simulink model "Backhoe_TiltCyl_Valve_Variants"  (R2020b)
settings: Solver=ode23t  StartTime=0.0  StopTime=60  MaxStep=0.01  RelTol=1e-3  EnableMultiTasking=on
PreLoadFcn:
  | Abstract=Simulink.Variant('ValveType4way==1');
  | Spool=Simulink.Variant('ValveType4way==2');
  | Nozzle_Center=Simulink.Variant('ValveType4way==3');
  | Nozzle_Feedback=Simulink.Variant('ValveType4way==4');
  | ValveType4way = 1;
  | 
  | warning('off','Simulink:Commands:LoadMdlParameterizedLink');
PostLoadFcn:
  | warning off Simulink:Engine:UsingDefaultMaxStepSize
  | warning off Simulink:blocks:MatchingFromNotFound
  | warning off Simulink:Engine:SaveWithParameterizedLinks_Warning
  | warning off Simulink:Engine:SolverMinStepNonlinearIterWarnForDAE
  | warning off Simulink:Commands:SetParamLinkChangeWarn
model workspace (MAT data in the model file):
  cylinderGray = [0.6 0.6 0.6]
  darkOrange = [0.8 0.5 0]
  glassBlue = [0.2 0.2 1]
  gray = [0.3 0.3 0.3]
  orange = [0.8 0.65 0]
  pistonGray = [0.4 0.4 0.4]
  rhoGlass = 2500
  rhoRubber = 1500
  rhoSteel = 7800
  tireBlack = [0.1 0.1 0.1]
  wheelGray = [0.6 0.6 0.6]
  yellow = [0.8 0.8 0]
undefined symbols (not defined in the file): BH_Param, sigbuilder_block, X, Y, Z
libraries: sm_lib x54, fl_lib x16, Backhoe_Lib x15, nesl_utility x8, sh_lib x6, Custom_Valve_Variants_Lib x3
(part 1 of 3)
CloseFcn:
  | try,close(h1_Backhoe_TiltCyl_Valve_Variants),end
  | clear h1_Backhoe_TiltCyl_Valve_Variants
  | try,close(h2_Backhoe_TiltCyl_Valve_Variants),end
  | clear h2_Backhoe_TiltCyl_Valve_Variants
  | try,close(h3_Backhoe_TiltCyl_Valve_Variants),end
  | clear h3_Backhoe_TiltCyl_Valve_Variants
  | try,close(h4_Backhoe_TiltCyl_Valve_Variants),end
  | clear h4_Backhoe_TiltCyl_Valve_Variants
  | 
  | clear simlog_Backhoe_TiltCyl_Valve_Variants
  | clear logsout_simlog_Backhoe_TiltCyl_Valve_Variants
Description:
  | Backhoe with Custom Valve
  | 
  | Copyright 2014-2020 The MathWorks, Inc.
settings Model: Creator=smiller  LastModifiedBy=smiller
settings DataIOCC: LimitDataPoints=on  SaveFormat=Array  ReturnWorkspaceOutputs=off
settings OptimizationCC: ExpressionDepthLimit=2147483647  LifeSpan=inf
settings DebuggingCC: UnderspecifiedInitializationDetection=Classic  MergeDetectMultiDrivingBlocksExec=none  SolverPrmCheckMsg=warning  AllowSymbolicDim=off  StateNameClashWarn=warning  PregeneratedLibrarySubsystemCodeDiagnostic=none  SFUnexpectedBacktrackingDiag=warning  SFNoUnconditionalDefaultTransitionDiag=warning  SFExecutionAtInitializationDiag=none  ArithmeticOperatorsInVariantConditions=warning
settings HardwareCC: ProdBitPerPointer=32  ProdBitPerSizeT=32  ProdBitPerPtrDiffT=32  ProdLargestAtomicFloat=None  ProdIntDivRoundTo=Undefined  ProdEndianess=Unspecified  ProdWordSize=32  ProdHWDeviceType=32-bit Generic
settings ModelReferenceCC: PropagateSignalLabelsOutOfModel=off
settings SFSimCC: SimUseLocalCustomCode=off  CustomCodeUndefinedFunction=UseInterfaceOnly
settings RTWCC: RTWUseLocalCustomCode=off
settings CodeAppCC: StateflowObjectComments=on
settings GRTTargetCC: TargetLangStandard=C89/C90 (ANSI)
settings ConfigComp: CovMetricSettings=dw  CovSaveCumulativeToWorkspaceVar=on  CovSaveSingleToWorkspaceVar=on  CovExternalEMLEnable=off  CovSFcnEnable=off
settings SimscapeCC: SimscapeNormalizeSystem=off  SimscapeLogType=all  SimscapeLogName=simlog_Backhoe_TiltCyl_Valve_Variants  SimscapeLogDataHistory=10000
settings ConfigurationSet: Description=SimMechanics 2G
settings ExplorerConfigSet: InternalSimMechanicsExplorerSettings="<ExplorerConfiguration><canonicalview>default</canonicalview><AnimationSetting><BasePlaybackSpeed>1.0</BasePlaybackSpeed><PlaybackSpeedFactor>1.0</PlaybackSpeedFactor></AnimationSetting><TilePanel><TileInfo><Tiles Columns=\"1\" Count=\"1\" Rows=\"1\"><Column Weight=\"1\"/><Row Weight=\"1\"/><Tile Height=\"1\" Width=\"1\" X=\"0\" Y=\"0\"/></Tiles></TileInfo><SceneInfo><SceneViewer><BGColor><R>1</R><G>1</G><B>1</B></BGColor><Camera><DoPerspective>off</DoPerspective><Position><X>0.528725759523142269</X><Y>-5.20390358957664034</Y><Z>-12.0546820877544469</Z></Position><Center><X>2.55521134765160207</X><Y>-1.1721933566146352</Y><Z>-0.0122773925518812436</Z></Center><Up><X>0.814497762035467865</X><Y>-0.577432689239198105</Y><Z>0.0562573109666866522</Z></Up><ViewLimDist>1</ViewLimDist><YLim>4.64006309682449647</YLim><XLim>7.37103468240321025</XLim></Camera></SceneViewer></SceneInfo></TilePanel><MechEditorPanel><Cameras/><GfxPanelCameraMap/><VideoCreator><PlaybackSpeedRatio>1.0</PlaybackSpeedRatio><FrameRate>30</FrameRate><VideoFormat>Motion JPEG AVI</VideoFormat><FrameSize>auto</FrameSize></VideoCreator></MechEditorPanel></ExplorerConfiguration>"

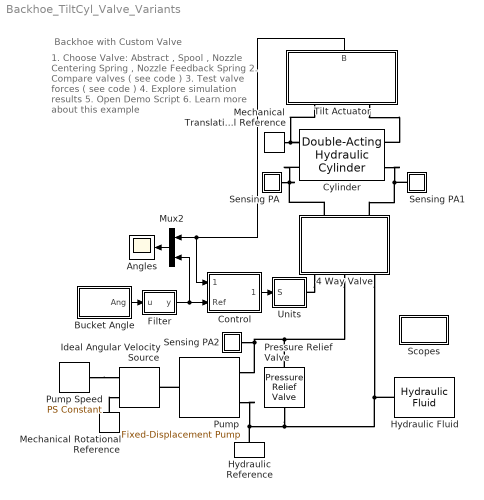
== system Backhoe_TiltCyl_Valve_Variants ==
  note: 1. Choose Valve: Abstract , Spool ,
      | Nozzle Centering Spring ,
      | Nozzle Feedback Spring
      | 2. Compare valves ( see code )
      | 3. Test valve forces ( see code )
      | 4. Explore simulation results
      | 5. Open Demo Script
      | 6. Learn more about this example
  note: Backhoe with Custom Valve
  4 Way Valve : Subsystem  InitFcn=|  BlockChoice=Servovalve_Flapper  Variant=on  mask(Four-Way Servovalve, Customizable){valvetype=Abstract, orifice_width=24.5, max_spool_travel=0.005, x0_orifice_PA=-1e-4, x0_orifice_PB=-1e-4, x0_orifice_AT=-1e-4, x0_orifice_BT=-1e-4, spool_mass=0.124, spool_damping=162, spool_rad_clear=0.05, spool_hyd_frc=Enable, x0_nozzle=0.5, max_nozzle_area=3.14, pump_spool_orifice_area=1, act_gain=250*10, act_timeconstant=1e-2, act_saturation=0.3}
      | %temp_maskObj = Simulink.Mask.get(gcb);
      | %temp_vt_h = temp_maskObj.getParameter('valvetype');
      | %set_param(gcb,'valvetype',temp_vt_h.TypeOptions{ValveType4way});
      mask prompts: valvetype "Valve Type"; orifice_width "Orifice Width (mm):"; max_spool_travel "Max Orifice Length (m):"; x0_orifice_PA "Initial Opening PA (mm):"; x0_orifice_PB "Initial Opening PB (mm):"; x0_orifice_AT "Initial Opening AT (mm):"; x0_orifice_BT "Initial Opening BT (mm):"; spool_mass "Spool Mass (kg):"; spool_damping "Centering Spring Damping (N/(m/s)):"; spool_rad_clear "Spool Radial Clearance (mm):"; spool_hyd_frc "Hydraulic Forces:"; x0_nozzle "Nozzle Initial Opening (mm):"; max_nozzle_area "Nozzle Max Area (mm^2):"; pump_spool_orifice_area "Pump Spool Orifice Area (mm):"; act_gain "Gain"; act_timeconstant "Time Constant (s)"; act_saturation "Saturation"
      mask help: Four-way servovalve with custom levels of fidelity. Configure spool actuation designs and dynamics below.
      mask init:
      | temp_maskObj = Simulink.Mask.get(gcb);
      | temp_vt_h = temp_maskObj.getParameter('valvetype');
      | temp_modeval = find(strcmp(temp_vt_h.Value,temp_vt_h.TypeOptions));
      | evalin('base',['ValveType4way = ' num2str(temp_modeval) ';']);
      | 
      | temp_orif_h = find_system(gcbh,...
      |     'regexp','on',...
      |     'SearchDepth', 1,...
      |     'LookUnderMasks','on',...
      |     'Parent', gcb,...
      |     'spool_hyd_frc','.*',...
      |     'VariantObject', get_param(gcb,'activevariant'));
      | 
      | if(~isempty(temp_orif_h))
      |     set_param(temp_orif_h,'spool_hyd_frc',...
      |         get_param(gcb,'spool_hyd_frc'));
      | end
      | 
      | clear temp_maskObj temp_vt_h temp_modeval
      settings: AttributesFormatString=%<ActiveVariant>
      mask TypeOptions valvetype: Abstract | Spool | Flapper Nozzle Centering Spring | Flapper Nozzle Feedback Spring
      mask Callback valvetype:
      | temp_maskObj = Simulink.Mask.get(gcb);
      | temp_vt_h = temp_maskObj.getParameter('valvetype');
      | temp_modeval = find(strcmp(get_param(gcb,'valvetype'),temp_vt_h.TypeOptions));
      | 
      | %disp(['VALVE MODE = ' num2str(temp_modeval)]);
      | 
      | temp_im_h = temp_maskObj.getDialogControl('valveimage');
      | temp_tabN_h = temp_maskObj.getDialogControl('TabNozzle');
      | temp_tabS_h = temp_maskObj.getDialogControl('TabSpool');
      | temp_tabA_h = temp_maskObj.getDialogControl('TabActuator');
      | 
      | if (temp_modeval == 1)
      |     temp_im_h.FilePath = 'Custom_Valve_Abstract_IMAGE.jpg';
      |     temp_tabS_h.Visible = 'off';
      |     temp_tabN_h.Visible = 'off';
      |     temp_tabA_h.Visible = 'on';
      | elseif (temp_modeval == 2)
      |     temp_im_h.FilePath = 'Custom_Valve_Spool_IMAGE.jpg';
      |     temp_tabS_h.Visible = 'on';
      |     temp_tabN_h.Visible = 'off';
      |     temp_tabA_h.Visible = 'off';
      | elseif (temp_modeval == 3)
      |     temp_im_h.FilePath = 'Custom_Valve_Flapper_Nozzle_Centering_Spring_IMAGE.jpg';
      |     temp_tabS_h.Visible = 'on';
      |     temp_tabN_h.Visible = 'on';
      |     temp_tabA_h.Visible = 'off';
      | else
      |     temp_im_h.FilePath = 'Custom_Valve_Flapper_Nozzle_Feedback_Spring_IMAGE.jpg';
      |     temp_tabS_h.Visible = 'on';
      |     temp_tabN_h.Visible = 'on';
      |     temp_tabA_h.Visible = 'off';
      | end
      | 
      | %disp(['FILE PATH = ' temp_im_h.FilePath]);
      | %disp(' ');
      | 
      | clear temp_maskObj temp_vt_h temp_modeval
      | clear temp_im_h temp_tabS_h temp_tabN_h
      mask TypeOptions spool_hyd_frc: Disable | Enable
      mask DialogControl TabValve Prompt: Valve
      mask DialogControl TabOrifice Prompt: Orifice
      mask DialogControl TabSpool Prompt: Spool
      mask DialogControl TabNozzle Prompt: Nozzle
      mask DialogControl TabActuator Prompt: Actuator
      mask Display:
      | blk = find_system(gcbh, 'SearchDepth', 1,'LookUnderMasks','on', 'Parent', gcb, 'VariantObject', get_param(gcb,'activevariant'));
      | eval(get_param(blk, 'MaskDisplay'));
  Angles : Scope
  Bucket Angle : Subsystem  Tag=STV Subsys  LoadFcn=sigbuilder_block('load');  StartFcn=sigbuilder_block('start');  StopFcn=sigbuilder_block('stop');  ClipboardFcn=sigbuilder_block('clipboard');  mask(Sigbuilder block){tuvar=[0:10]}
      mask help: Simulink:masks:SigbuilderBlock_MD
      mask init:
      | if ~strcmp(get_param(bdroot(gcbh),'SimulationStatus'),'stopped') tuvar = sigbuilder_block('maskInit'); end
      settings: CopyFcn=sigbuilder_block('copy');  DeleteFcn=sigbuilder_block('delete');  ModelCloseFcn=sigbuilder_block('modelClose');  PreSaveFcn=sigbuilder_block('preSave');  PauseFcn=sigbuilder_block('pause');  ContinueFcn=sigbuilder_block('continue');  NameChangeFcn=sigbuilder_block('namechange');  OpenFcn=sigbuilder_block('open',[267.6 46.8 624.6 408 ]);  CloseFcn=sigbuilder_block('close');
      mask Display: plot(0, 0, 100, 100,[2, 2, 32, 32, 2], [68, 8, 8, 68, 68],[32, 2], [38, 38], [32, 19, 2],[53, 60, 44], [32, 17, 17, 2],[16, 16, 31, 31]);txt = getActiveGroup(gcbh);text(2, 100, txt,'verticalAlignment', 'top');
  Control : Subsystem  mask(PID Controller){upperLim=10, lowerLim=-120, Kp=10, Ki=0.2, Kd=0.2, N=100}
      mask prompts: upperLim "Upper Limit [deg]"; lowerLim "Lower Limit [deg]"
      mask help: This block takes in a reference angle and measured angle, and uses a PID Controller with saturation to give a control command.
  Cylinder : sh_lib/Hydraulic Cylinders/Double-Acting Hydraulic Cylinder  Tag=Factory Generic  area_A=BH_Param.Tilt_Actuator.Cylinder.Area_A m^2  area_B=BH_Param.Tilt_Actuator.Cylinder.Area_B m^2  stroke=BH_Param.Tilt_Actuator.Cylinder.Stroke m  init_pos=BH_Param.Tilt_Actuator.Cylinder.x0 m  dead_vol_A=BH_Param.Tilt_Actuator.Cylinder.DeadVol_A m^3  dead_vol_B=BH_Param.Tilt_Actuator.Cylinder.DeadVol_B m^3  init_pressure_A=BH_Param.Tilt_Actuator.Cylinder.PA0 Pa  init_pressure_B=1.17e7 Pa  k_sh=1.4  stiff=1e+06 N/m  D=150 N/(m/s)  hardstop_model=3  transition=0.1 mm  or=2
      settings: SourceProductBaseCode=SH  InternalSimscapePortConfiguration="{\"Bottom\":[],\"Left\":[{\"id\":\"C\",\"label\":\"C\",\"type\":\"foundation.mechanical.translational.translational\"},{\"id\":\"A\",\"label\":\"A\",\"type\":\"foundation.hydraulic.hydraulic\"}],\"Right\":[{\"id\":\"R\",\"label\":\"R\",\"type\":\"foundation.mechanical.translational.translational\"},{\"id\":\"B\",\"label\":\"B\",\"type\":\"foundation.hydraulic.hydraulic\"}],\"Top\":[]}"
  Filter : Subsystem  mask{b=1e-1, x_initial=0}
      mask prompts: b "Filter time constant"; x_initial "Initial Output"
  Hydraulic Reference : fl_lib/Hydraulic/Hydraulic Elements/Hydraulic Reference
  Hydraulic Fluid : sh_lib/Hydraulic Utilities/Hydraulic Fluid  DataSource=1  SelFluid=9  SysTemp=50  TrapAir=0.004  ViscDerFactor=1  range_error=2
  Ideal Angular Velocity Source : fl_lib/Mechanical/Mechanical Sources/Ideal Angular Velocity Source
  Mechanical Rotational Reference : fl_lib/Mechanical/Rotational Elements/Mechanical Rotational Reference
  Mechanical Translational Reference : fl_lib/Mechanical/Translational Elements/Mechanical Translational Reference  Tag=Factory Generic
  Mux2 : Mux  Inputs=2
  Pressure Relief Valve : sh_lib/Valves/Pressure Control Valves/Pressure Relief Valve  valve_area_spec=1  p_diff_TLU=[30.15e5 : 15e3 : 31.35e5] Pa  area_TLU=[1 : 1 : 9] .* 1e-5 m^2  area_max=BH_Param.Hydraulic.PRV.Max_Area m^2  pres_set=BH_Param.Hydraulic.PRV.Pressure_Set Pa  reg_range=BH_Param.Hydraulic.PRV.Pressure_Rng Pa  C_d=BH_Param.Hydraulic.PRV.Flow_Disch_Coeff  A_leak=BH_Param.Hydraulic.PRV.Leakage_Area m^2  lam_spec=2  B_lam=0.999  Re_cr=BH_Param.Hydraulic.PRV.Re_Critical  dynamic=0  tau=0.1 s  area_init=1e-12 m^2
      settings: SourceProductBaseCode=SH  InternalSimscapePortConfiguration="{\"Bottom\":[],\"Left\":[{\"id\":\"A\",\"label\":\"A\",\"type\":\"foundation.hydraulic.hydraulic\"}],\"Right\":[{\"id\":\"B\",\"label\":\"B\",\"type\":\"foundation.hydraulic.hydraulic\"}],\"Top\":[]}"
  Pump : sh_lib/Pumps and Motors/Fixed-Displacement Pump  D=BH_Param.Hydraulic.Pump.Displacement m^3/rad  loss_spec=1  w_nominal=BH_Param.Hydraulic.Pump.Nominal_Ang_Vel rad/s  pr_nominal=BH_Param.Hydraulic.Pump.Nominal_Pressure Pa  visc_nominal=BH_Param.Hydraulic.Pump.Nominal_Kin_Visc cSt  dens_nominal=900 kg/m^3  efficiency_vol=BH_Param.Hydraulic.Pump.Vol_Eff  no_load_torque=0 N*m  torque_pressure_coeff=1*(BH_Param.Hydraulic.Pump.Displacement)*((BH_Param.Hydraulic.Pump.Vol_Eff)/(BH_Param.Hydraulic.Pump.Total_Eff)-1 ) N*m/Pa  p_diff_eff_TLU=[100000.0, 1000000.0, 2000000.0] Pa  omega_eff_TLU=[25.0, 50.0, 100.0, 200.0, 300.0, 400.0] rad/s  vol_eff_TLU=[0.816, 0.908, 0.954, 0.977, 0.981, 0.984; 0.325, 0.663, 0.831, 0.916, 0.925, 0.946; 0.137, 0.568, 0.78, 0.892, 0.893, 0.91]  mech_eff_TLU=[0.996, 0.996, 0.996, 0.996, 0.996, 0.996; 0.988, 0.989, 0.989, 0.989, 0.989, 0.99; 0.981, 0.981, 0.982, 0.982, 0.983, 0.984]  p_diff_loss_TLU=[100000.0, 1000000.0, 2000000.0] Pa  omega_loss_TLU=[25.0, 50.0, 100.0, 200.0, 300.0, 400.0] rad/s  vol_loss_TLU=[0.023, 0.023, 0.023, 0.023, 0.0285, 0.032; 0.0844, 0.0842, 0.0845, 0.084, 0.1125, 0.108; 0.1079, 0.108, 0.11, 0.108, 0.1605, 0.18] * 1e-3 m^3/s  mech_loss_TLU=[0.002, 0.002, 0.002, 0.002, 0.002, 0.002; 0.0607, 0.0556, 0.0556, 0.0556, 0.0556, 0.0505; 0.1937, 0.1937, 0.1833, 0.1833, 0.1729, 0.1626] N*m  pressure_threshold=1e5 Pa  omega_threshold=10 rad/s  quadrant_check=0  pressure_check=0  min_valid_pressure=0 Pa  vol_eff_min=1e-3  vol_eff_max=1  mech_eff_min=1e-3  mech_eff_max=1
      settings: SourceProductBaseCode=SH  InternalSimscapePortConfiguration="{\"Bottom\":[],\"Left\":[{\"id\":\"S\",\"label\":\"S\",\"type\":\"foundation.mechanical.rotational.rotational\"}],\"Right\":[{\"id\":\"P\",\"label\":\"P\",\"type\":\"foundation.hydraulic.hydraulic\"},{\"id\":\"T\",\"label\":\"T\",\"type\":\"foundation.hydraulic.hydraulic\"}],\"Top\":[]}"
  Pump Speed : fl_lib/Physical Signals/Sources/PS Constant  constant=188
  Scopes : Subsystem
  Sensing PA : Subsystem
      mask Display: disp('S')
  Sensing PA1 : Subsystem
      mask Display: disp('S')
  Sensing PA2 : Subsystem
      mask Display: disp('S')
  Tilt Actuator : Subsystem  Tag=PublishSubsystem
      mask Display:
      | image(imread('Backhoe_Tilt_Actuator_IMAGE.jpg'));
      | port_label('lconn',1,'C');
      | port_label('lconn',2,'R');
      | port_label('output',1,'B');
  Units : Subsystem
  wires:
  Tilt Actuator/1(B) -> Control/1(Meas), Mux2/1
  Control/1(Cmd) -> Units/1(S)
  Mux2/1 -> Angles/1
  Bucket Angle/1(Ang) -> Filter/1(u)
  Filter/1(y) -> Mux2/2, Control/2(Ref)
  connections:
  Pressure Relief Valve/LConn1 -- 4 Way Valve/RConn2 -- Pump/RConn1 -- Sensing PA2/LConn1
  Pump/RConn2 -- Hydraulic Reference/LConn1 -- Pressure Relief Valve/RConn1 -- 4 Way Valve/RConn3 -- Hydraulic Fluid/RConn1
  Mechanical Rotational Reference/LConn1 -- Ideal Angular Velocity Source/RConn2
  Pump/LConn1 -- Ideal Angular Velocity Source/LConn1
  Pump Speed/RConn1 -- Ideal Angular Velocity Source/RConn1
  Sensing PA1/LConn1 -- 4 Way Valve/LConn2 -- Cylinder/RConn2
  Tilt Actuator/LConn1 -- Mechanical Translational Reference/LConn1 -- Cylinder/LConn1
  Cylinder/LConn2 -- 4 Way Valve/LConn1 -- Sensing PA/LConn1
  Tilt Actuator/LConn2 -- Cylinder/RConn1
  4 Way Valve/RConn1 -- Units/RConn1

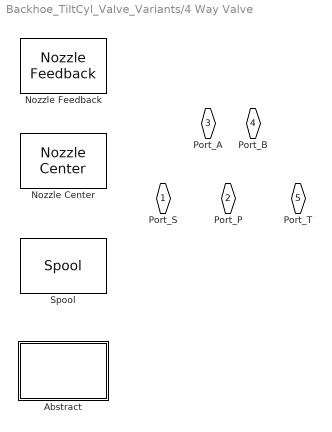
== system Backhoe_TiltCyl_Valve_Variants/4 Way Valve ==
  Abstract : Subsystem  Tag=PublishSubsystem  AncestorBlock=Custom_Valve_Variants_Lib/Abstract  VariantControl=Abstract  mask(Four-Way Valve){orifice_width=orifice_width, max_spool_travel=max_spool_travel, x0_orifice_PA=x0_orifice_PA, x0_orifice_PB=x0_orifice_PB, x0_orifice_AT=x0_orifice_AT, x0_orifice_BT=x0_orifice_BT, act_gain=act_gain, act_timeconstant=act_timeconstant, act_saturation=act_saturation}
      mask prompts: orifice_width "Orifice Width (mm):"; max_spool_travel "Max Orifice Length (m):"; x0_orifice_PA "Initial Opening PA (mm):"; x0_orifice_PB "Initial Opening PB (mm):"; x0_orifice_AT "Initial Opening AT (mm):"; x0_orifice_BT "Initial Opening BT (mm):"; act_gain "Gain"; act_timeconstant "Time Constant (s)"; act_saturation "Saturation"
      mask help: Four-way hydraulic directional valve.
      mask DialogControl ParameterTabVar0 Prompt: Orifice
      mask DialogControl Container4 Prompt: Actuator
      mask Display:
      | plot([0;337.311462499201;337.311462499201;0;0], [566.910021007061;566.910021007061;0;0;566.910021007061])
      | %hold on
      | plot([84.6585631370544;241.503668949008], [353;353])
      | plot([84.6585631370544;241.503668949008], [214;214])
      | plot([84.6585631370544;241.503668949008;241.503668949008;84.6585631370544;84.6585631370544], [491;491;76;76;491])
      | plot([84.6585631370544;241.503668949008], [449;449])
      | plot([241.503668949008;210.071657784283], [310;310])
      | plot([210.071657784283;210.071657784283;210.071657784283], [326;295;310.414731502533])
      | plot([241.503668949008;210.071657784283], [257;257])
      | plot([210.071657784283;210.071657784283;210.071657784283], [272;241;236.464468762279])
      | plot([84.6585631370544;115.964594297111], [257;257])
      | plot([115.964594297111;115.964594297111;115.964594297111], [272;241;236.464468762279])
      | plot([84.6585631370544;115.964594297111], [310;310])
      | plot([115.964594297111;115.964594297111;115.964594297111], [326;295;310.414731502533])
      | plot([84.6585631370544;241.503668949008], [185;110])
      | plot([241.503668949008;84.6585631370544], [185;110])
      | plot([84.6585631370544;241.503668949008], [395;395])
      | patch([85.0365031510592;110.547454096377;121.885654516518;85.0365031510592], [110;140;120;110], [0;0;0])
      | plot([85.0365031510592;110.547454096377;121.885654516518;85.0365031510592], [110;140;120;110])
      | patch([240.936758928001;204.087607562542;215.425807982683;240.936758928001], [109;120;140;109], [0;0;0])
      | plot([240.936758928001;204.087607562542;215.425807982683;240.936758928001], [109;120;140;109])
      | patch([83.6507230997086;127.554754726589;127.554754726589;83.6507230997086], [451;461;440;451], [0;0;0])
      | plot([83.6507230997086;127.554754726589;127.554754726589;83.6507230997086], [451;461;440;451])
      | patch([245.283069089055;201.253057457507;201.253057457507;245.283069089055], [394;405;384;394], [0;0;0])
      | plot([245.283069089055;201.253057457507;201.253057457507;245.283069089055], [394;405;384;394])
      | 
      | color('red');
      | port_label('LConn', 1,'A')
      | port_label('LConn', 2,'B')
      | port_label('RConn', 1,'S')
      | port_label('RConn', 2,'P')
      | port_label('RConn', 3,'T')
  Nozzle Center : Custom_Valve_Variants_Lib/Nozzle Center  Tag=PublishSubsystem  VariantControl=Nozzle_Center  orifice_width=orifice_width  max_spool_travel=max_spool_travel  x0_orifice_PA=x0_orifice_PA  x0_orifice_PB=x0_orifice_PB  x0_orifice_AT=x0_orifice_AT  x0_orifice_BT=x0_orifice_BT  spool_mass=spool_mass  ctr_spr_stiffness=360000  spool_damping=spool_damping*2  spool_rad_clear=spool_rad_clear  spool_hyd_frc=Enable  x0_nozzle=x0_nozzle  max_nozzle_area=max_nozzle_area  pump_spool_orifice_area=pump_spool_orifice_area
      link override Valve/Orifices: OverrideUsingVariant=With_Force
  Nozzle Feedback : Custom_Valve_Variants_Lib/Nozzle Feedback  Tag=PublishSubsystem  VariantControl=Nozzle_Feedback  orifice_width=orifice_width  max_spool_travel=max_spool_travel  x0_orifice_PA=x0_orifice_PA  x0_orifice_PB=x0_orifice_PB  x0_orifice_AT=x0_orifice_AT  x0_orifice_BT=x0_orifice_BT  spool_mass=spool_mass  spool_damping=spool_damping  spool_rad_clear=spool_rad_clear  spool_hyd_frc=Enable  x0_nozzle=x0_nozzle  max_nozzle_area=max_nozzle_area  pump_spool_orifice_area=pump_spool_orifice_area
  Spool : Custom_Valve_Variants_Lib/Spool  Tag=PublishSubsystem  VariantControl=Spool  orifice_width=orifice_width  max_spool_travel=max_spool_travel  x0_orifice_PA=x0_orifice_PA  x0_orifice_PB=x0_orifice_PB  x0_orifice_AT=x0_orifice_AT  x0_orifice_BT=x0_orifice_BT  spool_mass=spool_mass  ctr_spr_stiffness=36000*100  spool_damping=spool_damping*20  spool_rad_clear=spool_rad_clear  spool_hyd_frc=Enable
  Port_S : PMIOPort  Side=Right
  Port_P : PMIOPort  Port=2  Side=Right
  Port_A : PMIOPort  Port=3  Side=Left
  Port_B : PMIOPort  Port=4  Side=Left
  Port_T : PMIOPort  Port=5  Side=Right

== system Backhoe_TiltCyl_Valve_Variants/Bucket Angle ==
  Demux : Demux  Tag=STV Demux  Outputs=1
      settings: DisplayOption=none
  FromWs : FromWorkspace  Tag=STV FromWs  VariableName=tuvar  OutputAfterFinalValue=Holding final value
      SigBuilderData=|
      | common.afterFinalStr = 'Hold final value'
      | common.sampleTime = '0'
      | dataSet.timeRange = [0 60]
      | dataSet.name = 'Ref'
      | sbobj.Groups.Name = 'Ref'
      | sbobj.Groups.Signals.Name = 'Ang'
      | sbobj.Groups.Signals.XData = [0 7 11 24 28.5 40 42 51.5 53.5 60]
      | sbobj.Groups.Signals.YData = [0 0 -90 -90 0 0 -110 -110 0 0]
      | sbobj.Groups.TimeRange = [0 60]
  Ang : Outport  Tag=STV Outport  VectorParamsAs1DForOutWhenUnconnected=off
  wires:
  Demux/1 -> Ang/1
  FromWs/1 -> Demux/1

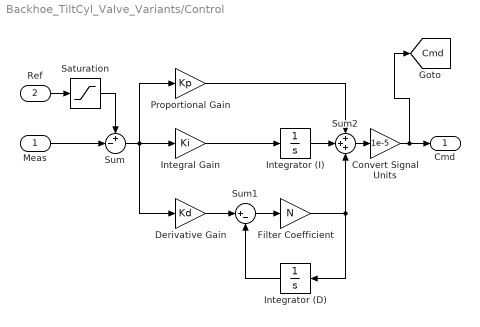
== system Backhoe_TiltCyl_Valve_Variants/Control ==
  Meas : Inport
  Ref : Inport  Port=2
  Convert Signal Units : Gain  Gain=1e-5
  Derivative Gain : Gain  Gain=Kd
  Filter Coefficient : Gain  Gain=N
  Integral Gain : Gain  Gain=Ki
  Integrator (D) : Integrator
  Integrator (I) : Integrator
  Proportional Gain : Gain  Gain=Kp
  Saturation : Saturate  UpperLimit=upperLim  LowerLimit=lowerLim
  Sum : Sum  Inputs=+-|
  Sum1 : Sum  Inputs=|+-
  Sum2 : Sum  Inputs=+++
  Cmd : Outport  VectorParamsAs1DForOutWhenUnconnected=off
  tag scope: Cmd=global
  wires:
  Saturation/1 -> Sum/1
  Meas/1 -> Sum/2
  Ref/1 -> Saturation/1
  Sum/1 -> Integral Gain/1, Proportional Gain/1, Derivative Gain/1
  Sum2/1 -> Convert Signal Units/1
  Integrator (I)/1 -> Sum2/2
  Integrator (D)/1 -> Sum1/2
  Filter Coefficient/1 -> Integrator (D)/1, Sum2/3
  Sum1/1 -> Filter Coefficient/1
  Derivative Gain/1 -> Sum1/1
  Integral Gain/1 -> Integrator (I)/1
  Proportional Gain/1 -> Sum2/1
  Convert Signal Units/1 -> [Cmd], Cmd/1

== system Backhoe_TiltCyl_Valve_Variants/Filter ==
  u : Inport
  Gain : Gain  Gain=1/b
  Integrator : Integrator  InitialCondition=x_initial
  Sum : Sum  Inputs=|+-
  y : Outport  VectorParamsAs1DForOutWhenUnconnected=off
  wires:
  Gain/1 -> Integrator/1
  Integrator/1 -> y/1, Sum/2
  u/1 -> Sum/1
  Sum/1 -> Gain/1

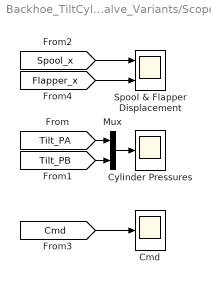
== system Backhoe_TiltCyl_Valve_Variants/Scopes ==
  Cmd : Scope
  Cylinder Pressures : Scope
  Mux : Mux  Inputs=2
  Spool & Flapper Displacement : Scope  NumInputPorts=2
  wires:
  [Spool_x] -> Spool & Flapper Displacement/1
  [Flapper_x] -> Spool & Flapper Displacement/2
  [Tilt_PB] -> Mux/2
  [Tilt_PA] -> Mux/1
  Mux/1 -> Cylinder Pressures/1
  [Cmd] -> Cmd/1

== system Backhoe_TiltCyl_Valve_Variants/Sensing PA ==
  Hydraulic Pressure Sensor : fl_lib/Hydraulic/Hydraulic Sensors/Hydraulic Pressure Sensor
  Hydraulic Reference1 : fl_lib/Hydraulic/Hydraulic Elements/Hydraulic Reference
  PS-Simulink Converter1 : nesl_utility/PS-Simulink Converter  PhysicalDomain=network_engine_domain  SubClassName=ps_output  LeftPortType=input  RightPortType=output  PseudoPeriodic=off  Frequencies=[]  Unit=1  AffineConversion=off
  A : PMIOPort  Side=Left
  tag scope: Tilt_PA=global
  wires:
  PS-Simulink Converter1/1 -> [Tilt_PA]
  connections:
  PS-Simulink Converter1/LConn1 -- Hydraulic Pressure Sensor/RConn2
  Hydraulic Reference1/LConn1 -- Hydraulic Pressure Sensor/RConn1
  Hydraulic Pressure Sensor/LConn1 -- A/RConn1

== system Backhoe_TiltCyl_Valve_Variants/Sensing PA1 ==
  Hydraulic Pressure Sensor : fl_lib/Hydraulic/Hydraulic Sensors/Hydraulic Pressure Sensor
  Hydraulic Reference1 : fl_lib/Hydraulic/Hydraulic Elements/Hydraulic Reference
  PS-Simulink Converter1 : nesl_utility/PS-Simulink Converter  PhysicalDomain=network_engine_domain  SubClassName=ps_output  LeftPortType=input  RightPortType=output  PseudoPeriodic=off  Frequencies=[]  Unit=1  AffineConversion=off
  A : PMIOPort  Side=Left
  tag scope: Tilt_PB=global
  wires:
  PS-Simulink Converter1/1 -> [Tilt_PB]
  connections:
  Hydraulic Pressure Sensor/LConn1 -- A/RConn1
  Hydraulic Reference1/LConn1 -- Hydraulic Pressure Sensor/RConn1
  PS-Simulink Converter1/LConn1 -- Hydraulic Pressure Sensor/RConn2

== system Backhoe_TiltCyl_Valve_Variants/Sensing PA2 ==
  Hydraulic Pressure Sensor : fl_lib/Hydraulic/Hydraulic Sensors/Hydraulic Pressure Sensor
  Hydraulic Reference1 : fl_lib/Hydraulic/Hydraulic Elements/Hydraulic Reference
  PS-Simulink Converter1 : nesl_utility/PS-Simulink Converter  PhysicalDomain=network_engine_domain  SubClassName=ps_output  LeftPortType=input  RightPortType=output  PseudoPeriodic=off  Frequencies=[]  Unit=1  AffineConversion=off
  A : PMIOPort  Side=Left
  tag scope: Lift_PP=global
  wires:
  PS-Simulink Converter1/1 -> [Lift_PP]
  connections:
  PS-Simulink Converter1/LConn1 -- Hydraulic Pressure Sensor/RConn2
  Hydraulic Reference1/LConn1 -- Hydraulic Pressure Sensor/RConn1
  Hydraulic Pressure Sensor/LConn1 -- A/RConn1

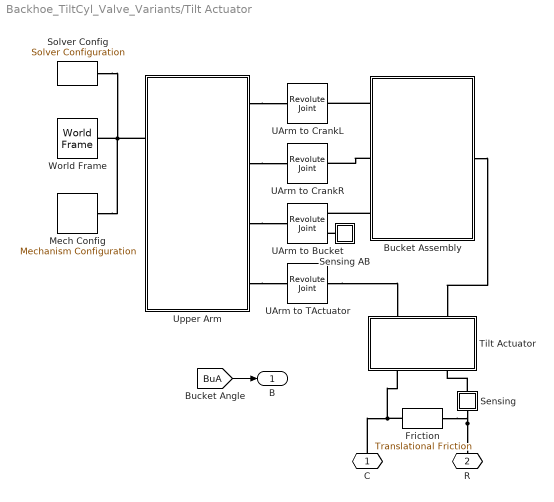
== system Backhoe_TiltCyl_Valve_Variants/Tilt Actuator ==
  Bucket Assembly : Subsystem
      mask Display:
      | image(imread('Backhoe_Arm_Bucket_Asy_IMAGE.JPG'));
      | port_label('lconn',1,'UAL');
      | port_label('lconn',2,'UAR');
      | port_label('lconn',3,'UA');
      | port_label('rconn',1,'TAct');
  Friction : fl_lib/Mechanical/Translational Elements/Translational Friction  brkwy_frc=BH_Param.Tilt_Actuator.Friction.Breakaway N  brkwy_vel=0.060623 m/s  Col_frc=BH_Param.Tilt_Actuator.Friction.Coulomb N  visc_coef=BH_Param.Tilt_Actuator.Friction.Viscous N/(m/s)  v_specify=off  v_priority=High  v=0 m/s  v_nominal_specify=off  v_nominal_unit=m/s  v_nominal_value=1  f_specify=off  f_priority=High  f=0 N  f_nominal_specify=off  f_nominal_unit=N  f_nominal_value=1
      settings: SourceProductBaseCode=SS  InternalSimscapePortConfiguration="{\"Bottom\":[],\"Left\":[{\"id\":\"R\",\"label\":\"R\",\"type\":\"foundation.mechanical.translational.translational\"}],\"Right\":[{\"id\":\"C\",\"label\":\"C\",\"type\":\"foundation.mechanical.translational.translational\"}],\"Top\":[]}"
  Mech Config : sm_lib/Utilities/Mechanism Configuration  UniformGravity=Constant  GravityVector=[0 -9.81 0]  GravityVectorUnits=m/s^2  GravityUnits=m/s^2  LinearizationDelta=0.001  JointModeTransitionNonlinearIterations=2
  Sensing : Subsystem
      mask Display: disp('S')
  Sensing AB : Subsystem
      mask Display: disp('S')
  Solver Config : nesl_utility/Solver Configuration  PhysicalDomain=network_engine_domain  SubClassName=solver  LeftPortType=input  RightPortType=generic  Tones=[]  Harmonics=[]  SimulateNoise=off  Profile=off  UseLocalSampling=off  EnableSwitchedLinearOptims=on  FrequencyDomain=off  UseCCode=off  RelTol=0.001  AbsTol=1e-06  MinStep=1e-09  ToWorkspace=off  RevertToSquareIcSolve=off  NumHomotopyIterations=100  PhasorMode=off  PhasorModeNumHarmonics=1  DoDC=off  ResidualTolerance=1e-9  UseLocalSolver=off  LocalSolverChoice=NE_BACKWARD_EULER_ADVANCER  LocalSolverSampleTime=.001  DoFixedCost=off  MaxNonlinIter=3  MaxModeIter=2  ComputeImpulses=off  ImpulseIterations=2  LinearAlgebra=Sparse  EquationFormulation=NE_TIME_EF  DelaysMemoryBudget=1024  AutomaticFiltering=on  FilteringTimeConstant=0.001  PartitionStorageMethod=AS_NEEDED  PartitionMemoryBudget=1024  PartitionMethod=FAST
  Tilt Actuator : Subsystem  mask(Hydraulic Actuator){Lcyl=1.9, Rcyl=0.2, Lpist=1.9, Rpist=0.12, Lbase=0.65, Wbase=0.425, Rbp=0.075, Lbp=0.8, Whead=0.35, Lhead=0.65, Rhp=0.075, Lhp=0.9, circlePoints=25, cylColor=BH_Param.Colors.cylinderGray, rhoCyl=BH_Param.Densities.rhoSteel, pistColor=BH_Param.Colors.pistonGray, rhoPist=BH_Param.Densities.rhoSteel, connColor=BH_Param.Colors.gray, rhoConn=BH_Param.Densities.rhoSteel}
      mask prompts: Lcyl "Lcyl [m]"; Rcyl "Rcyl [m]"; Lpist "Lpist [m]"; Rpist "Rpist [m]"; Lbase "Lbase [m]"; Wbase "Wbase [m]"; Rbp "Rbp [m]"; Lbp "Lbp [m]"; Whead "Whead [m]"; Lhead "Lhead [m]"; Rhp "Rhp [m]"; Lhp "Lhp [m]"; circlePoints "Circle Mesh Resolution"; cylColor "Cylinder Color"; rhoCyl "Cylinder Density [kg/m^3]"; pistColor "Piston Color"; rhoPist "Piston Density [kg/m^3]"; connColor "Connector Color"; rhoConn "Connector Density [kg/m^3]"
      mask help:
      | Consists of the backhoe hydraulic actuator assembly.
      |
      | Zero piston displacement corresponds to the piston and cylinder centers of mass in the same position. Positive piston displacement is outward motion, and negative piston displacement is inward motion.
      |
      | Attachment points are:
      | C: Center of the Cylinder base bracket hole.
      | H: Center of the Piston Head bracket hole.
      | Both attachment points are configured for Revolute joints.
      |
      | The Simulink Signal input port supplies a Pressure value P (in Pa) to a Simscape hydraulic network.
      |
      | Click on Help to view a schematic of the hydraulic actuator, its configurable dimension parameters and attachment points (in red).
      mask init:
      | % Hollow Cylinder cross-section
      | cylSection = [];
      | 
      | for i = 0:2*circlePoints
      |     angle = (i/circlePoints)*pi;
      |     cylSection = [cylSection; Rcyl*cos(angle) Rcyl*sin(angle)];
      | end
      | 
      | for i = 0:2*circlePoints
      |     angle = -(i/circlePoints)*pi;
      |     cylSection = [cylSection; Rpist*cos(angle) Rpist*sin(angle)];
      | end
      mask Help: web('Backhoe_Actuator.html');
      mask Display:
      | image(imread('Backhoe_Arm_Actuator_IMAGE.jpg'));
      | port_label('lconn',1,'R');
      | port_label('lconn',2,'C');
      | port_label('rconn',1,'Cr');
      | port_label('rconn',2,'UA');
      | %port_label('input',1,'Cmd');
  UArm to Bucket : sm_lib/Joints/Revolute Joint  JointMode=Normal  SenseConstraintForce=off  SenseConstraintForceX=off  SenseConstraintForceY=off  SenseConstraintForceZ=off  SenseConstraintTorque=off  SenseConstraintTorqueX=off  SenseConstraintTorqueY=off  SenseConstraintTorqueZ=off  SenseTotalForce=off  SenseTotalForceX=off  SenseTotalForceY=off  SenseTotalForceZ=off  SenseTotalTorque=off  SenseTotalTorqueX=off  SenseTotalTorqueY=off  SenseTotalTorqueZ=off  CompositeWrenchDir=FollowerOnBase  CompositeWrenchFrame=BaseFrame  EquilibriumPosition=0  EquilibriumPositionUnits=deg  SpringStiffness=0  SpringStiffnessUnits=N*m/deg  DampingCoefficient=0  DampingCoefficientUnits=N*m/(deg/s)  TorqueActuationMode=NoTorque  MotionActuationMode=ComputedMotion  SensePosition=on  SenseVelocity=off  SenseAcceleration=off  SenseTorqueForce=off  SenseLowerLimitTorqueForce=off  SenseUpperLimitTorqueForce=off  LowerLimitSpecify=off  LowerLimitBound=-90  LowerLimitBoundUnits=deg  LowerLimitStiffness=1e4  LowerLimitStiffnessUnits=N*m/deg  LowerLimitDamping=10  LowerLimitDampingUnits=N*m/(deg/s)  LowerLimitTransitionRegionWidth=0.1  LowerLimitTransitionRegionWidthUnits=deg  UpperLimitSpecify=off  UpperLimitBound=90  UpperLimitBoundUnits=deg  UpperLimitStiffness=1e4  UpperLimitStiffnessUnits=N*m/deg  UpperLimitDamping=10  UpperLimitDampingUnits=N*m/(deg/s)  UpperLimitTransitionRegionWidth=0.1  UpperLimitTransitionRegionWidthUnits=deg  PositionTargetSpecify=on  PositionTargetPriority=High  PositionTargetValue=0  PositionTargetValueUnits=deg  VelocityTargetSpecify=off  VelocityTargetPriority=High  VelocityTargetValue=0  VelocityTargetValueUnits=deg/s
  UArm to CrankL : sm_lib/Joints/Revolute Joint  JointMode=Normal  SenseConstraintForce=off  SenseConstraintForceX=off  SenseConstraintForceY=off  SenseConstraintForceZ=off  SenseConstraintTorque=off  SenseConstraintTorqueX=off  SenseConstraintTorqueY=off  SenseConstraintTorqueZ=off  SenseTotalForce=off  SenseTotalForceX=off  SenseTotalForceY=off  SenseTotalForceZ=off  SenseTotalTorque=off  SenseTotalTorqueX=off  SenseTotalTorqueY=off  SenseTotalTorqueZ=off  CompositeWrenchDir=FollowerOnBase  CompositeWrenchFrame=BaseFrame  EquilibriumPosition=0  EquilibriumPositionUnits=deg  SpringStiffness=0  SpringStiffnessUnits=N*m/deg  DampingCoefficient=0  DampingCoefficientUnits=N*m/(deg/s)  TorqueActuationMode=NoTorque  MotionActuationMode=ComputedMotion  SensePosition=off  SenseVelocity=off  SenseAcceleration=off  SenseTorqueForce=off  SenseLowerLimitTorqueForce=off  SenseUpperLimitTorqueForce=off  LowerLimitSpecify=off  LowerLimitBound=-90  LowerLimitBoundUnits=deg  LowerLimitStiffness=1e4  LowerLimitStiffnessUnits=N*m/deg  LowerLimitDamping=10  LowerLimitDampingUnits=N*m/(deg/s)  LowerLimitTransitionRegionWidth=0.1  LowerLimitTransitionRegionWidthUnits=deg  UpperLimitSpecify=off  UpperLimitBound=90  UpperLimitBoundUnits=deg  UpperLimitStiffness=1e4  UpperLimitStiffnessUnits=N*m/deg  UpperLimitDamping=10  UpperLimitDampingUnits=N*m/(deg/s)  UpperLimitTransitionRegionWidth=0.1  UpperLimitTransitionRegionWidthUnits=deg  PositionTargetSpecify=off  PositionTargetPriority=Low  PositionTargetValue=-150  PositionTargetValueUnits=deg  VelocityTargetSpecify=off  VelocityTargetPriority=High  VelocityTargetValue=0  VelocityTargetValueUnits=deg/s
  UArm to CrankR : sm_lib/Joints/Revolute Joint  JointMode=Normal  SenseConstraintForce=off  SenseConstraintForceX=off  SenseConstraintForceY=off  SenseConstraintForceZ=off  SenseConstraintTorque=off  SenseConstraintTorqueX=off  SenseConstraintTorqueY=off  SenseConstraintTorqueZ=off  SenseTotalForce=off  SenseTotalForceX=off  SenseTotalForceY=off  SenseTotalForceZ=off  SenseTotalTorque=off  SenseTotalTorqueX=off  SenseTotalTorqueY=off  SenseTotalTorqueZ=off  CompositeWrenchDir=FollowerOnBase  CompositeWrenchFrame=BaseFrame  EquilibriumPosition=0  EquilibriumPositionUnits=deg  SpringStiffness=0  SpringStiffnessUnits=N*m/deg  DampingCoefficient=0  DampingCoefficientUnits=N*m/(deg/s)  TorqueActuationMode=NoTorque  MotionActuationMode=ComputedMotion  SensePosition=off  SenseVelocity=off  SenseAcceleration=off  SenseTorqueForce=off  SenseLowerLimitTorqueForce=off  SenseUpperLimitTorqueForce=off  LowerLimitSpecify=off  LowerLimitBound=-90  LowerLimitBoundUnits=deg  LowerLimitStiffness=1e4  LowerLimitStiffnessUnits=N*m/deg  LowerLimitDamping=10  LowerLimitDampingUnits=N*m/(deg/s)  LowerLimitTransitionRegionWidth=0.1  LowerLimitTransitionRegionWidthUnits=deg  UpperLimitSpecify=off  UpperLimitBound=90  UpperLimitBoundUnits=deg  UpperLimitStiffness=1e4  UpperLimitStiffnessUnits=N*m/deg  UpperLimitDamping=10  UpperLimitDampingUnits=N*m/(deg/s)  UpperLimitTransitionRegionWidth=0.1  UpperLimitTransitionRegionWidthUnits=deg  PositionTargetSpecify=off  PositionTargetPriority=High  PositionTargetValue=0  PositionTargetValueUnits=deg  VelocityTargetSpecify=off  VelocityTargetPriority=High  VelocityTargetValue=0  VelocityTargetValueUnits=deg/s
  UArm to TActuator : sm_lib/Joints/Revolute Joint  JointMode=Normal  SenseConstraintForce=off  SenseConstraintForceX=off  SenseConstraintForceY=off  SenseConstraintForceZ=off  SenseConstraintTorque=off  SenseConstraintTorqueX=off  SenseConstraintTorqueY=off  SenseConstraintTorqueZ=off  SenseTotalForce=off  SenseTotalForceX=off  SenseTotalForceY=off  SenseTotalForceZ=off  SenseTotalTorque=off  SenseTotalTorqueX=off  SenseTotalTorqueY=off  SenseTotalTorqueZ=off  CompositeWrenchDir=FollowerOnBase  CompositeWrenchFrame=BaseFrame  EquilibriumPosition=0  EquilibriumPositionUnits=deg  SpringStiffness=0  SpringStiffnessUnits=N*m/deg  DampingCoefficient=0  DampingCoefficientUnits=N*m/(deg/s)  TorqueActuationMode=NoTorque  MotionActuationMode=ComputedMotion  SensePosition=off  SenseVelocity=off  SenseAcceleration=off  SenseTorqueForce=off  SenseLowerLimitTorqueForce=off  SenseUpperLimitTorqueForce=off  LowerLimitSpecify=off  LowerLimitBound=-90  LowerLimitBoundUnits=deg  LowerLimitStiffness=1e4  LowerLimitStiffnessUnits=N*m/deg  LowerLimitDamping=10  LowerLimitDampingUnits=N*m/(deg/s)  LowerLimitTransitionRegionWidth=0.1  LowerLimitTransitionRegionWidthUnits=deg  UpperLimitSpecify=off  UpperLimitBound=90  UpperLimitBoundUnits=deg  UpperLimitStiffness=1e4  UpperLimitStiffnessUnits=N*m/deg  UpperLimitDamping=10  UpperLimitDampingUnits=N*m/(deg/s)  UpperLimitTransitionRegionWidth=0.1  UpperLimitTransitionRegionWidthUnits=deg  PositionTargetSpecify=on  PositionTargetPriority=Low  PositionTargetValue=-90  PositionTargetValueUnits=deg  VelocityTargetSpecify=off  VelocityTargetPriority=High  VelocityTargetValue=0  VelocityTargetValueUnits=deg/s
  Upper Arm : Subsystem
      mask Display:
      | image(imread('Backhoe_Arm_Upper_IMAGE.JPG'));
      | port_label('lconn',1,'LA');
      | port_label('lconn',2,'RAct');
      | port_label('rconn',1,'CrL');
      | port_label('rconn',2,'CrR');
      | port_label('rconn',3,'B');
      | port_label('rconn',4,'TAct');
  World Frame : sm_lib/Frames and Transforms/World Frame
  C : PMIOPort  Side=Left
  R : PMIOPort  Port=2  Side=Left
  B : Outport  VectorParamsAs1DForOutWhenUnconnected=off
  wires:
  [BuA] -> B/1
  connections:
  C/RConn1 -- Tilt Actuator/LConn2 -- Friction/RConn1
  Bucket Assembly/LConn1 -- UArm to CrankL/RConn1
  Sensing AB/LConn1 -- UArm to Bucket/RConn2
  Upper Arm/RConn1 -- UArm to CrankL/LConn1
  Upper Arm/RConn4 -- UArm to TActuator/LConn1
  Upper Arm/RConn2 -- UArm to CrankR/LConn1
  Bucket Assembly/LConn2 -- UArm to CrankR/RConn1
  Bucket Assembly/RConn1 -- Tilt Actuator/RConn1
  Friction/LConn1 -- Sensing/LConn1 -- R/RConn1
  UArm to TActuator/RConn1 -- Tilt Actuator/RConn2
  Bucket Assembly/LConn3 -- UArm to Bucket/RConn1
  Upper Arm/RConn3 -- UArm to Bucket/LConn1
  Mech Config/RConn1 -- Upper Arm/LConn1 -- Solver Config/RConn1 -- World Frame/RConn1
  Sensing/RConn1 -- Tilt Actuator/LConn1

== system Backhoe_TiltCyl_Valve_Variants/Units ==
  S : Inport
  Simulink-PS Converter : nesl_utility/Simulink-PS Converter  PhysicalDomain=network_engine_domain  SubClassName=ps_input  LeftPortType=input  RightPortType=output  PseudoPeriodic=off  Frequencies=[]  NoiseDistribution=none  NoiseParameters=[]  Unit=m  AffineConversion=off  FilteringAndDerivatives=zero  SimscapeFilterOrder=1  InputFilterTimeConstant=0.005  UdotUserProvided=0
  PS : PMIOPort  Side=Right
  wires:
  S/1 -> Simulink-PS Converter/1
  connections:
  Simulink-PS Converter/RConn1 -- PS/RConn1

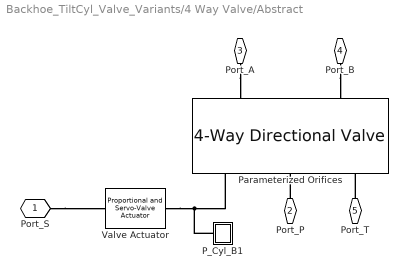
== system Backhoe_TiltCyl_Valve_Variants/4 Way Valve/Abstract ==
  P_Cyl_B1 : Subsystem
  Parameterized Orifices : sh_lib/Valves/Directional Valves/4-Way Directional Valve  area_spec=1  x_0_P_A=x0_orifice_PA mm  x_0_P_B=x0_orifice_PB mm  x_0_A_T=x0_orifice_AT mm  x_0_B_T=x0_orifice_BT mm  mdl_type_identical=1  mdl_type_different=1  opening_max=max_spool_travel m  area_max=orifice_width*max_spool_travel*1e3 mm^2  opening_max_P_A=0.005 m  area_max_P_A=0.5e-4 m^2  opening_max_P_B=0.005 m  area_max_P_B=0.5e-4 m^2  opening_max_A_T=0.005 m  area_max_A_T=0.5e-4 m^2  opening_max_B_T=0.005 m  area_max_B_T=0.5e-4 m^2  opening_area_tab="[  -0.002 0 0.002 0.005 0.015 ] m"  area_tab="[  1e-09 2.0352e-07 4.0736e-05 0.00011438 0.00034356 ] m^2"  opening_flow_rate_tab="[  -0.002 0 0.002 0.005 0.015 ] m"  pressure_tab="[  -1e+07 -5e+06 -2e+06 2e+06 5e+06 1e+07 ] Pa"  flow_rate_tab="[  -1e-07 -7.0711e-08 -4.4721e-08 4.4721e-08 7.0711e-08 1e-07 ; -2.0352e-05 -1.4391e-05 -9.1017e-06 9.1017e-06 1.4391e-05 2.0352e-05 ; -0.0040736 -0.0028805 -0.0018218 0.0018218 0.0028805 0.0040736 ; -0.011438 -0.0080879 -0.0051152 0.0051152 0.0080879 0.011438 ; -0.034356 -0.024293 -0.015364 0.015364 0.024293 0.034356 ; ] m^3/s"  opening_area_tab_P_A=[-0.002, 0.0, 0.002, 0.005, 0.015] m  area_tab_P_A=[1.0e-9, 2.0352e-7, 4.0736e-5, 0.00011438, 0.00034356] m^2  opening_flow_rate_tab_P_A=[-0.002, 0.0, 0.002, 0.005, 0.015] m  pressure_tab_P_A=[-10000000.0, -5000000.0, -2000000.0, 2000000.0, 5000000.0, 10000000.0] Pa  flow_rate_tab_P_A=[-1.0e-7, -7.0711e-8, -4.4721e-8, 4.4721e-8, 7.0711e-8, 1.0e-7; -2.0352e-5, -1.4391e-5, -9.1017e-6, 9.1017e-6, 1.4391e-5, 2.0352e-5; -0.0040736, -0.0028805, -0.0018218, 0.0018218, 0.0028805, 0.0040736; -0.011438, -0.0080879, -0.0051152, 0.0051152, 0.0080879, 0.011438; -0.034356, -0.024293, -0.015364, 0.015364, 0.024293, 0.034356] m^3/s  opening_area_tab_P_B=[-0.002, 0.0, 0.002, 0.005, 0.015] m  area_tab_P_B=[1.0e-9, 2.0352e-7, 4.0736e-5, 0.00011438, 0.00034356] m^2  opening_flow_rate_tab_P_B=[-0.002, 0.0, 0.002, 0.005, 0.015] m  pressure_tab_P_B=[-10000000.0, -5000000.0, -2000000.0, 2000000.0, 5000000.0, 10000000.0] Pa  flow_rate_tab_P_B=[-1.0e-7, -7.0711e-8, -4.4721e-8, 4.4721e-8, 7.0711e-8, 1.0e-7; -2.0352e-5, -1.4391e-5, -9.1017e-6, 9.1017e-6, 1.4391e-5, 2.0352e-5; -0.0040736, -0.0028805, -0.0018218, 0.0018218, 0.0028805, 0.0040736; -0.011438, -0.0080879, -0.0051152, 0.0051152, 0.0080879, 0.011438; -0.034356, -0.024293, -0.015364, 0.015364, 0.024293, 0.034356] m^3/s  opening_area_tab_A_T=[-0.002, 0.0, 0.002, 0.005, 0.015] m  area_tab_A_T=[1.0e-9, 2.0352e-7, 4.0736e-5, 0.00011438, 0.00034356] m^2  opening_flow_rate_tab_A_T=[-0.002, 0.0, 0.002, 0.005, 0.015] m  pressure_tab_A_T=[-10000000.0, -5000000.0, -2000000.0, 2000000.0, 5000000.0, 10000000.0] Pa  flow_rate_tab_A_T=[-1.0e-7, -7.0711e-8, -4.4721e-8, 4.4721e-8, 7.0711e-8, 1.0e-7; -2.0352e-5, -1.4391e-5, -9.1017e-6, 9.1017e-6, 1.4391e-5, 2.0352e-5; -0.0040736, -0.0028805, -0.0018218, 0.0018218, 0.0028805, 0.0040736; -0.011438, -0.0080879, -0.0051152, 0.0051152, 0.0080879, 0.011438; -0.034356, -0.024293, -0.015364, 0.015364, 0.024293, 0.034356] m^3/s  opening_area_tab_B_T=[-0.002, 0.0, 0.002, 0.005, 0.015] m  area_tab_B_T=[1.0e-9, 2.0352e-7, 4.0736e-5, 0.00011438, 0.00034356] m^2  opening_flow_rate_tab_B_T=[-0.002, 0.0, 0.002, 0.005, 0.015] m  pressure_tab_B_T=[-10000000.0, -5000000.0, -2000000.0, 2000000.0, 5000000.0, 10000000.0] Pa  flow_rate_tab_B_T=[-1.0e-7, -7.0711e-8, -4.4721e-8, 4.4721e-8, 7.0711e-8, 1.0e-7; -2.0352e-5, -1.4391e-5, -9.1017e-6, 9.1017e-6, 1.4391e-5, 2.0352e-5; -0.0040736, -0.0028805, -0.0018218, 0.0018218, 0.0028805, 0.0040736; -0.011438, -0.0080879, -0.0051152, 0.0051152, 0.0080879, 0.011438; -0.034356, -0.024293, -0.015364, 0.015364, 0.024293, 0.034356] m^3/s  interp_method_identical=1  interp_method_different=1  extrap_method_identical=1  extrap_method_different=1  A_leak=1e-12 m^2  C_d=0.7  lam_spec=2  B_lam=0.999  Re_cr=12
      settings: SourceProductBaseCode=SH  InternalSimscapePortConfiguration="{\"Bottom\":[],\"Left\":[{\"id\":\"A\",\"label\":\"A\",\"type\":\"foundation.hydraulic.hydraulic\"},{\"id\":\"B\",\"label\":\"B\",\"type\":\"foundation.hydraulic.hydraulic\"}],\"Right\":[{\"id\":\"S\",\"label\":\"S\",\"type\":\"input\"},{\"id\":\"P\",\"label\":\"P\",\"type\":\"foundation.hydraulic.hydraulic\"},{\"id\":\"T\",\"label\":\"T\",\"type\":\"foundation.hydraulic.hydraulic\"}],\"Top\":[]}"
  Valve Actuator : sh_lib/Valves/Valve Actuators/Proportional and Servo-Valve Actuator  gain=act_gain  time_constant=act_timeconstant s  saturation=act_saturation
      settings: SourceProductBaseCode=SH  InternalSimscapePortConfiguration="{\"Bottom\":[],\"Left\":[{\"id\":\"I\",\"label\":\"\",\"type\":\"input\"}],\"Right\":[{\"id\":\"O\",\"label\":\"\",\"type\":\"output\"}],\"Top\":[]}"
  Port_S : PMIOPort  Side=Right
  Port_P : PMIOPort  Port=2  Side=Right
  Port_A : PMIOPort  Port=3  Side=Left
  Port_B : PMIOPort  Port=4  Side=Left
  Port_T : PMIOPort  Port=5  Side=Right
  connections:
  Port_A/RConn1 -- Parameterized Orifices/LConn1
  Port_B/RConn1 -- Parameterized Orifices/LConn2
  Valve Actuator/RConn1 -- P_Cyl_B1/LConn1 -- Parameterized Orifices/RConn1
  Port_P/RConn1 -- Parameterized Orifices/RConn2
  Port_T/RConn1 -- Parameterized Orifices/RConn3
  Port_S/RConn1 -- Valve Actuator/LConn1
